simulink model "Simulation"  (R2012b)
settings: Solver=FixedStepDiscrete  StartTime=0.0  StopTime=500  FixedStep=0.1  RelTol=1e-3
settings Model: Creator=Kerianne  LastModifiedBy=Kerianne
settings DataIOCC: SaveFormat=Structure
settings OptimizationCC: InlineParams=on
settings ModelReferenceCC: ModelDependencies=|
  | % Specify the model dependencies as a cell array of file names.  The dependencies
  | % automatically include the model and linked library files.  For files
  | % not on the MATLAB path, use absolute paths; prefix $MDL to a file path if the
  | % path is relative to the location of the model file; wildcards are allowed; use a '%'
  | % to comment out a line; use '...' to continue lines.  For example,
  | %
  | % {'D:\Work\parameters.mat', '$MDL\mdlvars.mat', ...
  | % 'D:\Work\masks\*.m'}
  | constants.m

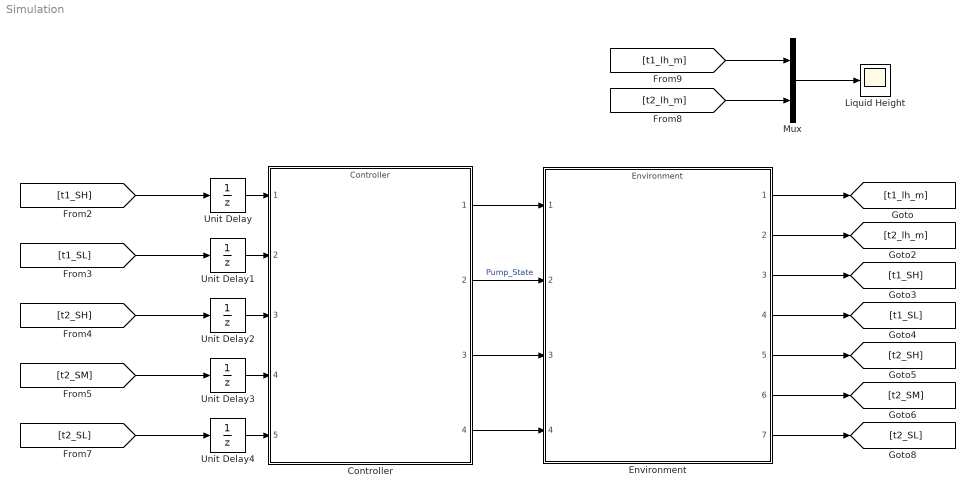
== system Simulation ==
  Controller : ModelReference  ModelNameDialog=Controller  SimulationMode=Normal  ModelReferenceVersion=1.19  CopyOfModelName=Controller  DefaultDataLogging=on
  Environment : ModelReference  ModelNameDialog=Environment  SimulationMode=Normal  ModelReferenceVersion=1.47  CopyOfModelName=Environment  DefaultDataLogging=on
  Liquid Height : Scope
  Mux : Mux  Inputs=2
  Unit Delay{,1..4} (5 alike) : UnitDelay  SampleTime=-1
  wires:
  Controller/1 -> Environment/1
  Controller/2 -> Environment/2  "Pump_State"
  Controller/3 -> Environment/3
  Controller/4 -> Environment/4
  [t1_SL] -> Unit Delay1/1
  [t2_SM] -> Unit Delay3/1
  [t1_SH] -> Unit Delay/1
  [t2_SH] -> Unit Delay2/1
  [t2_SL] -> Unit Delay4/1
  Environment/7 -> [t2_SL]
  Environment/6 -> [t2_SM]
  Environment/5 -> [t2_SH]
  Environment/4 -> [t1_SL]
  Environment/3 -> [t1_SH]
  Environment/2 -> [t2_lh_m]
  Environment/1 -> [t1_lh_m]
  [t1_lh_m] -> Mux/1
  [t2_lh_m] -> Mux/2
  Mux/1 -> Liquid Height/1
  Unit Delay/1 -> Controller/1
  Unit Delay1/1 -> Controller/2
  Unit Delay2/1 -> Controller/3
  Unit Delay3/1 -> Controller/4
  Unit Delay4/1 -> Controller/5
